simulink library "Lib_Turbo_SFCCalc_TMATS"  (R2019b)
settings: Solver=ode45  StartTime=0.0  StopTime=10.0  RelTol=1e-3  EnableMultiTasking=on
Description:
  | Thomas Modules
settings Model: Creator=jwchapm2  LastModifiedBy=bhisma
settings DataIOCC: LimitDataPoints=on  SaveFormat=Array  ReturnWorkspaceOutputs=off
settings OptimizationCC: ExpressionDepthLimit=2147483647  LifeSpan=inf
settings DebuggingCC: UnderspecifiedInitializationDetection=Classic  MergeDetectMultiDrivingBlocksExec=none  SolverPrmCheckMsg=warning  StateNameClashWarn=warning  SFUnexpectedBacktrackingDiag=warning  SFNoUnconditionalDefaultTransitionDiag=warning  SFExecutionAtInitializationDiag=none  ArithmeticOperatorsInVariantConditions=warning
settings HardwareCC: ProdBitPerPointer=32  ProdBitPerSizeT=32  ProdBitPerPtrDiffT=32  ProdLargestAtomicFloat=None  ProdIntDivRoundTo=Undefined  ProdEndianess=Unspecified  ProdWordSize=32  ProdHWDeviceType=32-bit Generic
settings ModelReferenceCC: PropagateSignalLabelsOutOfModel=off
settings SFSimCC: SimUseLocalCustomCode=off  CustomCodeUndefinedFunction=UseInterfaceOnly
settings RTWCC: RTWUseLocalCustomCode=off
settings CodeAppCC: StateflowObjectComments=on
settings GRTTargetCC: TargetLangStandard=C89/C90 (ANSI)  GeneratePreprocessorConditionals=Disable all
settings ConfigComp: CovMetricSettings=dw  CovHtmlReporting=on  CovSaveCumulativeToWorkspaceVar=on  CovSaveSingleToWorkspaceVar=on  CovExternalEMLEnable=off

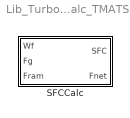
== system Lib_Turbo_SFCCalc_TMATS ==
  SFCCalc : Subsystem  mask(TMATS: SFC Calculation Library Block){}
      mask help: This block calculates specific fuel consumption (SFC) and net thrust (Fnet).
      mask Help: web(which('Turbo_TMATS_SFC.html'),'-helpbrowser')

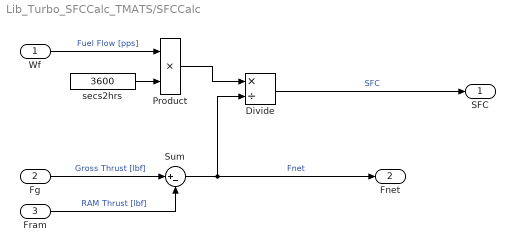
== system Lib_Turbo_SFCCalc_TMATS/SFCCalc ==
  Wf : Inport
  Fg : Inport  Port=2
  Fram : Inport  Port=3
  Divide : Product  Inputs=*/
  Product : Product
  Sum : Sum  Inputs=|+-
  secs2hrs : Constant  Value=3600
  SFC : Outport
  Fnet : Outport  Port=2
  wires:
  Fram/1 -> Sum/2  "RAM Thrust [lbf]"
  secs2hrs/1 -> Product/2
  Fg/1 -> Sum/1  "Gross Thrust [lbf]"
  Product/1 -> Divide/1
  Wf/1 -> Product/1  "Fuel Flow [pps]"
  Divide/1 -> SFC/1  "SFC"
  Sum/1 -> Divide/2, Fnet/1  "Fnet"
